simulink model "QUAD_EULER_MPC_SMC"  (R2024b)
settings: Solver=VariableStepAuto  StartTime=0.0  StopTime=10.0  RelTol=1e-3
values from neighbouring files (symbols this model uses):
  F1 = F1 + 2*(PSI_I'*C'*Q_z*C*PHI_I)    [Setup_MPC_SMC_Drone.m]
  F1_xy = F1_xy + 2*(PSI_xy_I'*C_xy'*Q_xy*C_xy*PHI_xy_I)    [Setup_MPC_SMC_Drone.m]
  F2 = F2 - 2*(PSI_I'*C'*Q_z*pi_n)    [Setup_MPC_SMC_Drone.m]
  F2_xy = F2_xy - 2*(PSI_xy_I'*C_xy'*Q_xy*pi_n)    [Setup_MPC_SMC_Drone.m]
  F3 = F3 - 2*(pi_nu'*Qt_z)    [Setup_MPC_SMC_Drone.m]
  F3_xy = F3_xy - 2*(pi_nu'*R_xy)    [Setup_MPC_SMC_Drone.m]
  F4 = F4 + 2*(PSI_I'*C'*Qt_z*C*SumG)    [Setup_MPC_SMC_Drone.m]
  g = 9.81    [Setup_MPC_SMC_Drone.m]
  G = [0;-g]    [Setup_MPC_SMC_Drone.m]
  H = H + 2*(PSI_I'*C'*Q_z*C*PSI_I + pi_nu'*Qt_z*pi_nu)    [Setup_MPC_SMC_Drone.m]
  H_xy = H_xy + 2*(PSI_xy_I'*C_xy'*Q_xy*C_xy*PSI_xy_I + pi_nu'*R_xy*pi_nu)    [Setup_MPC_SMC_Drone.m]
  J = diag([Jxx Jyy Jzz])    [Setup_MPC_SMC_Drone.m]
  m = 1.121    [Setup_MPC_SMC_Drone.m]
  N = 10    [Setup_MPC_SMC_Drone.m]
  N_xy = 10    [Setup_MPC_SMC_Drone.m]
  ny = size(C,1)    [Setup_MPC_SMC_Drone.m]
  ny_xy = size(C_xy,1)    [Setup_MPC_SMC_Drone.m]
  u_des = 0    [Setup_MPC_SMC_Drone.m]
  u_des_xy = [0;0]    [Setup_MPC_SMC_Drone.m]
undefined symbols (not defined in the file or in its folder): nu
libraries: matrix_library x1, aerolibutil x1
settings Model: Creator=Jorge  LastModifiedBy=Jorge

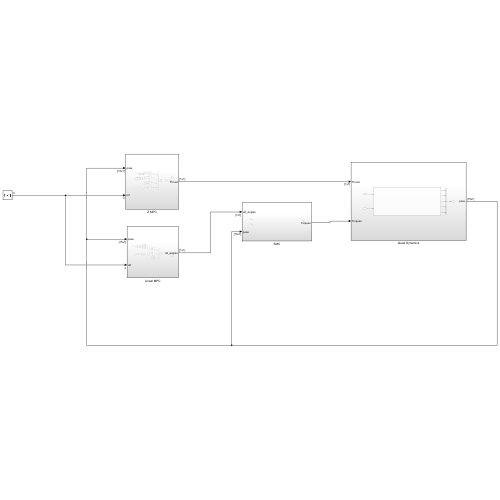
[thumbnail: Simulink's stored preview of the top-level diagram]
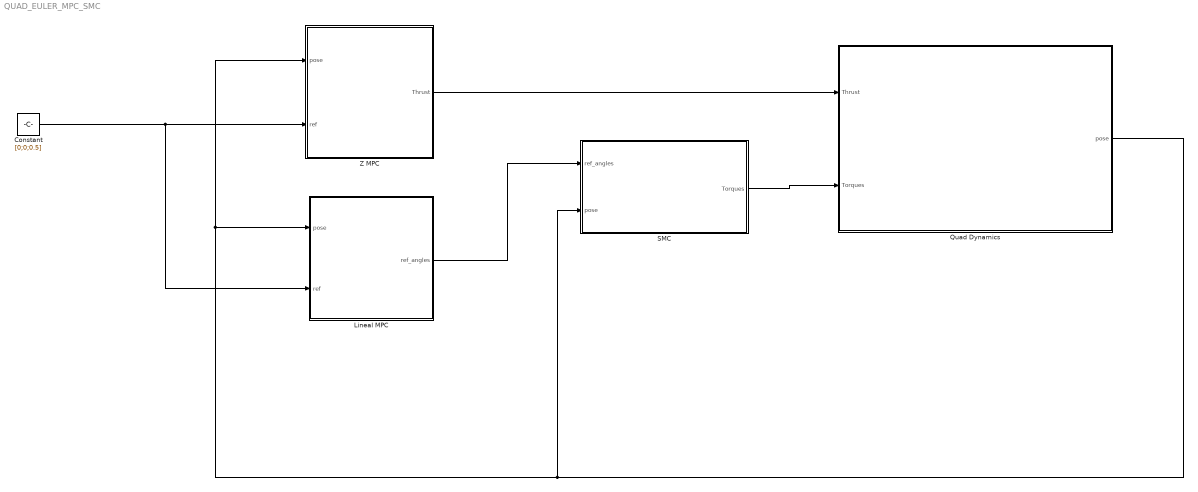
== system QUAD_EULER_MPC_SMC ==
  Constant : Constant  Value=[0;0;0.5]
  Lineal MPC : Subsystem
  Quad Dynamics : Subsystem
  SMC : Subsystem
  Z MPC : Subsystem
  wires:
  Quad Dynamics/1(pose) -> SMC/2(pose), Lineal MPC/1(pose), Z MPC/1(pose)
  Z MPC/1(Thrust) -> Quad Dynamics/1(Thrust)
  Constant/1 -> Lineal MPC/2(ref), Z MPC/2(ref)
  Lineal MPC/1(ref_angles) -> SMC/1(ref_angles)
  SMC/1(Torques) -> Quad Dynamics/2(Torques)

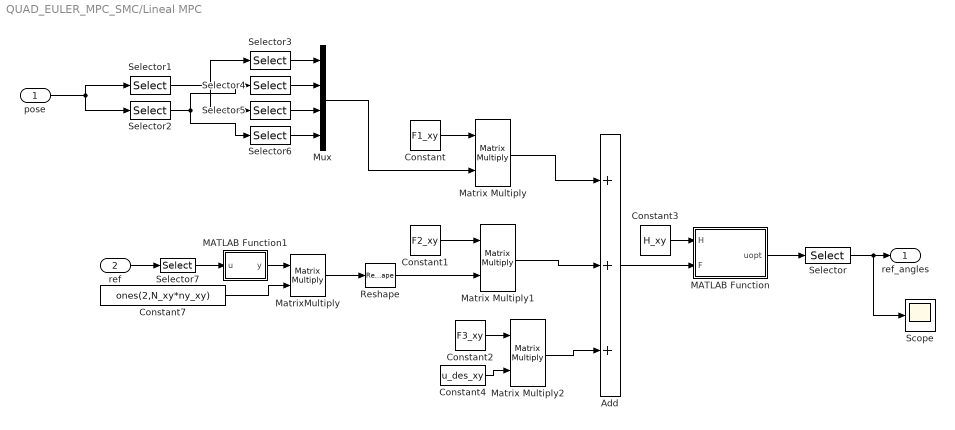
== system QUAD_EULER_MPC_SMC/Lineal MPC ==
  pose : Inport
  ref : Inport  Port=2
  Add : Sum  Inputs=+++
  Constant : Constant  Value=F1_xy
  Constant1 : Constant  Value=F2_xy
  Constant2 : Constant  Value=F3_xy
  Constant3 : Constant  Value=H_xy
  Constant4 : Constant  Value=u_des_xy
  Constant7 : Constant  Value=ones(2,N_xy*ny_xy)
  MATLAB Function : MATLAB Function  TreatAsAtomicUnit=on
  MATLAB Function1 : MATLAB Function  TreatAsAtomicUnit=on
  Matrix Multiply : Product  Multiplication=Matrix(*)
  Matrix Multiply1 : Product  Multiplication=Matrix(*)
  Matrix Multiply2 : Product  Multiplication=Matrix(*)
  MatrixMultiply : Product  Multiplication=Matrix(*)
  Mux : Mux
  Reshape : Reshape  OutputDimensionality=Customize  OutputDimensions=[N_xy*ny_xy,1]
  Scope : Scope
  Selector : Selector  InputPortWidth=20  IndexOptions=Index vector (dialog)  Indices=1  OutputSizes=1
  Selector1 : Selector  InputPortWidth=15  IndexOptions=Index vector (dialog)  Indices=[1 2]  OutputSizes=1
  Selector2 : Selector  InputPortWidth=15  IndexOptions=Index vector (dialog)  Indices=[4 5]  OutputSizes=1
  Selector3 : Selector  InputPortWidth=2  IndexOptions=Index vector (dialog)  Indices=1  OutputSizes=1
  Selector4 : Selector  InputPortWidth=2  IndexOptions=Index vector (dialog)  Indices=1  OutputSizes=1
  Selector5 : Selector  InputPortWidth=2  IndexOptions=Index vector (dialog)  Indices=2  OutputSizes=1
  Selector6 : Selector  InputPortWidth=2  IndexOptions=Index vector (dialog)  Indices=1  OutputSizes=1
  Selector7 : Selector  InputPortWidth=3  IndexOptions=Index vector (dialog)  Indices=[1:2]  OutputSizes=1
  ref_angles : Outport
  wires:
  Constant3/1 -> MATLAB Function/1(H)
  Add/1 -> MATLAB Function/2(F)
  MATLAB Function/1(uopt) -> Selector/1
  Selector/1 -> Scope/1, ref_angles/1
  pose/1 -> Selector2/1, Selector1/1
  Selector1/1 -> Selector3/1, Selector5/1
  Selector2/1 -> Selector4/1, Selector6/1
  Selector3/1 -> Mux/1
  Selector4/1 -> Mux/2
  Selector5/1 -> Mux/3
  Selector6/1 -> Mux/4
  Constant/1 -> Matrix Multiply/1
  Mux/1 -> Matrix Multiply/2
  Matrix Multiply/1 -> Add/1
  Matrix Multiply1/1 -> Add/2
  Constant1/1 -> Matrix Multiply1/1
  Constant7/1 -> MatrixMultiply/2
  ref/1 -> Selector7/1
  MatrixMultiply/1 -> Reshape/1
  Reshape/1 -> Matrix Multiply1/2
  Matrix Multiply2/1 -> Add/3
  Constant2/1 -> Matrix Multiply2/1
  Constant4/1 -> Matrix Multiply2/2
  Selector7/1 -> MATLAB Function1/1(u)
  MATLAB Function1/1(y) -> MatrixMultiply/1

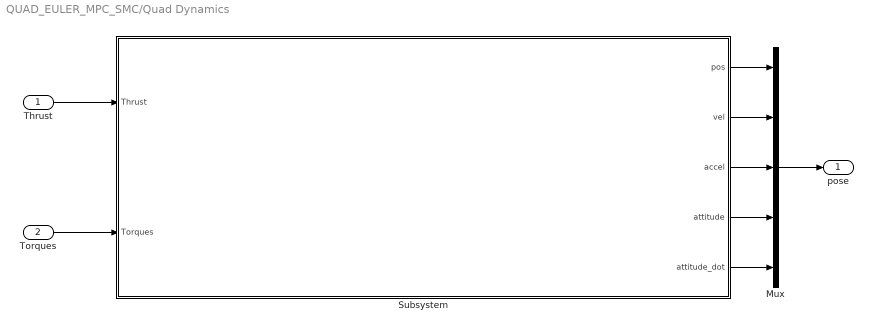
== system QUAD_EULER_MPC_SMC/Quad Dynamics ==
  Thrust : Inport
  Torques : Inport  Port=2
  Mux : Mux  Inputs=5
  Subsystem : Subsystem
  pose : Outport
  wires:
  Subsystem/1(pos) -> Mux/1
  Subsystem/2(vel) -> Mux/2
  Subsystem/3(accel) -> Mux/3
  Subsystem/4(attitude) -> Mux/4
  Subsystem/5(attitude_dot) -> Mux/5
  Thrust/1 -> Subsystem/1(Thrust)
  Torques/1 -> Subsystem/2(Torques)
  Mux/1 -> pose/1

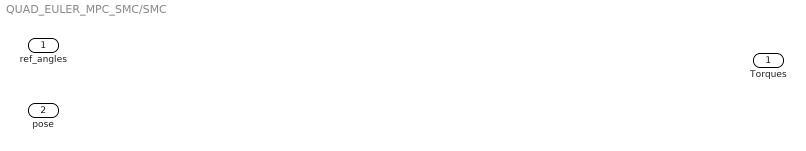
== system QUAD_EULER_MPC_SMC/SMC ==
  ref_angles : Inport
  pose : Inport  Port=2
  Torques : Outport

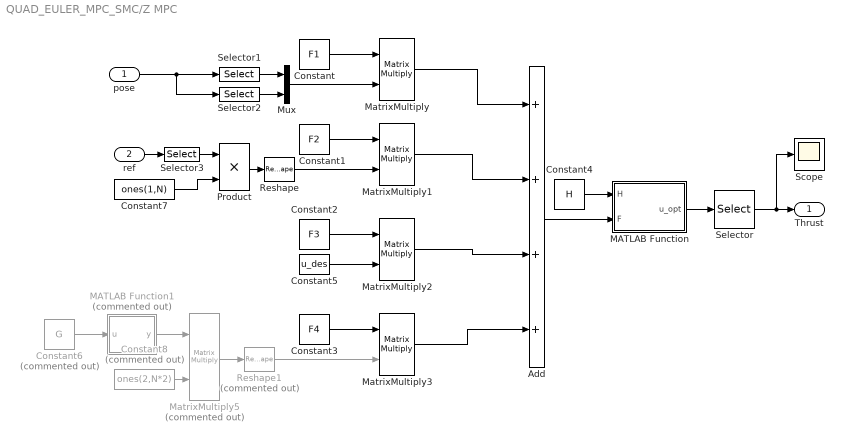
== system QUAD_EULER_MPC_SMC/Z MPC ==
  pose : Inport
  ref : Inport  Port=2
  Add : Sum  Inputs=++++
  Constant : Constant  Value=F1
  Constant1 : Constant  Value=F2
  Constant2 : Constant  Value=F3
  Constant3 : Constant  Value=F4
  Constant4 : Constant  Value=H
  Constant5 : Constant  Value=u_des
  Constant6 : Constant  Commented=on  Value=G
  Constant7 : Constant  Value=ones(1,N)
  Constant8 : Constant  Commented=on  Value=ones(2,N*2)
  MATLAB Function : MATLAB Function  TreatAsAtomicUnit=on
  MATLAB Function1 : MATLAB Function  Commented=on  TreatAsAtomicUnit=on
  MatrixMultiply{,1..3} (4 alike) : Product  Multiplication=Matrix(*)
  MatrixMultiply5 : Product  Commented=on  Multiplication=Matrix(*)
  Mux : Mux  Inputs=2
  Product : Product
  Reshape : Reshape  OutputDimensionality=Customize  OutputDimensions=[N*ny,1]
  Reshape1 : Reshape  Commented=on  OutputDimensionality=Customize  OutputDimensions=[2*N,1]
  Scope : Scope
  Selector : Selector  InputPortWidth=N*nu  IndexOptions=Index vector (dialog)  Indices=1  OutputSizes=1
  Selector1 : Selector  InputPortWidth=15  IndexOptions=Index vector (dialog)  Indices=3  OutputSizes=1
  Selector2 : Selector  InputPortWidth=15  IndexOptions=Index vector (dialog)  Indices=6  OutputSizes=1
  Selector3 : Selector  InputPortWidth=3  IndexOptions=Index vector (dialog)  Indices=3  OutputSizes=1
  Thrust : Outport
  wires:
  Add/1 -> MATLAB Function/2(F)
  Constant4/1 -> MATLAB Function/1(H)
  MATLAB Function/1(u_opt) -> Selector/1
  Selector/1 -> Scope/1, Thrust/1
  Constant/1 -> MatrixMultiply/1
  MatrixMultiply/1 -> Add/1
  MatrixMultiply1/1 -> Add/2
  MatrixMultiply2/1 -> Add/3
  MatrixMultiply3/1 -> Add/4
  Mux/1 -> MatrixMultiply/2
  Selector2/1 -> Mux/2
  Selector1/1 -> Mux/1
  pose/1 -> Selector2/1, Selector1/1
  Constant1/1 -> MatrixMultiply1/1
  Constant5/1 -> MatrixMultiply2/2
  Constant2/1 -> MatrixMultiply2/1
  ref/1 -> Selector3/1
  Constant7/1 -> Product/2
  Selector3/1 -> Product/1
  Product/1 -> Reshape/1
  Reshape/1 -> MatrixMultiply1/2
  Constant8/1 -> MatrixMultiply5/2
  Constant6/1 -> MATLAB Function1/1(u)
  MatrixMultiply5/1 -> Reshape1/1
  Reshape1/1 -> MatrixMultiply3/2
  Constant3/1 -> MatrixMultiply3/1
  MATLAB Function1/1(y) -> MatrixMultiply5/1

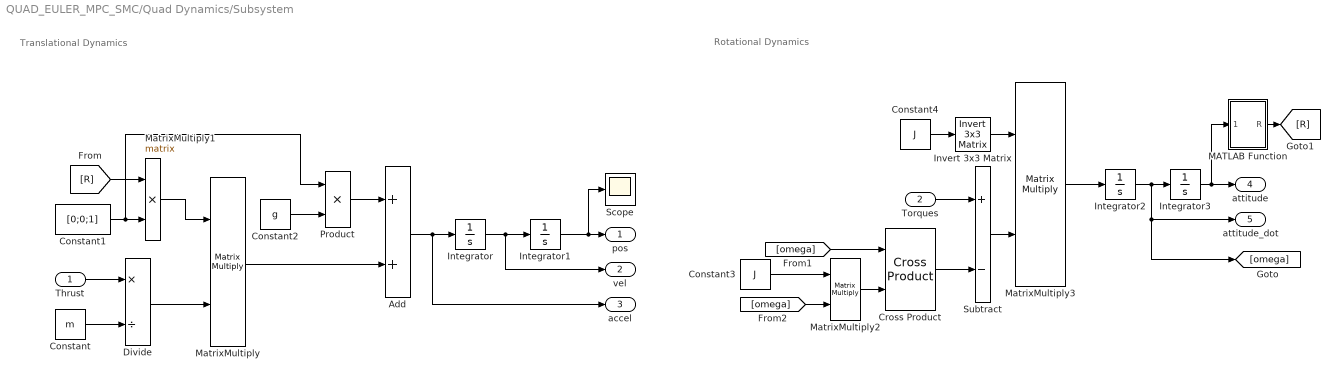
== system QUAD_EULER_MPC_SMC/Quad Dynamics/Subsystem ==
  note: Rotational Dynamics
  note: Translational Dynamics
  Thrust : Inport
  Torques : Inport  Port=2
  Add : Sum
  Constant : Constant  Value=m
  Constant1 : Constant  Value=[0;0;1]
  Constant2 : Constant  Value=g
  Constant3 : Constant  Value=J
  Constant4 : Constant  Value=J
  Cross Product : matrix_library/Cross Product
  Divide : Product  Inputs=*/
  Integrator{,1..3} (4 alike) : Integrator
  Invert 3x3 Matrix : aerolibutil/Invert  3x3 Matrix
  MATLAB Function : MATLAB Function  TreatAsAtomicUnit=on
  MatrixMultiply{,1..3} (4 alike) : Product  Multiplication=Matrix(*)
  Product : Product
  Scope : Scope
  Subtract : Sum  Inputs=+-
  pos : Outport
  vel : Outport  Port=2
  accel : Outport  Port=3
  attitude : Outport  Port=4
  attitude_dot : Outport  Port=5
  wires:
  Constant/1 -> Divide/2
  MatrixMultiply1/1 -> MatrixMultiply/1
  Integrator2/1 -> [omega], attitude_dot/1, Integrator3/1
  Constant2/1 -> Product/2
  Integrator1/1 -> Scope/1, pos/1
  Integrator/1 -> vel/1, Integrator1/1
  Constant4/1 -> Invert 3x3 Matrix/1
  [omega] -> Cross Product/1
  Constant3/1 -> MatrixMultiply2/1
  [omega] -> MatrixMultiply2/2
  Cross Product/1 -> Subtract/2
  Divide/1 -> MatrixMultiply/2
  Torques/1 -> Subtract/1
  [R] -> MatrixMultiply1/1
  MatrixMultiply/1 -> Add/2
  Integrator3/1 -> MATLAB Function/1(att), attitude/1
  MATLAB Function/1(R) -> [R]
  Constant1/1 -> Product/1, MatrixMultiply1/2
  MatrixMultiply3/1 -> Integrator2/1
  Add/1 -> accel/1, Integrator/1
  MatrixMultiply2/1 -> Cross Product/2
  Subtract/1 -> MatrixMultiply3/2
  Thrust/1 -> Divide/1
  Product/1 -> Add/1
  Invert 3x3 Matrix/1 -> MatrixMultiply3/1

== matlab function QUAD_EULER_MPC_SMC/Lineal MPC/MATLAB Function ==
  data: H input; uopt output; F input
function uopt = fcn(H,F)

uopt = -H\F;

== matlab function QUAD_EULER_MPC_SMC/Z MPC/MATLAB Function1 ==
  data: u input; y output
function y = fcn(u)

y = [u(1) u(2)];

== matlab function QUAD_EULER_MPC_SMC/Quad Dynamics/Subsystem/MATLAB Function ==
  data: att input; R output
function R = fcn(att)
phi = att(1);
theta = att(2);
psi = att(3);

R = [
cos(psi)*cos(theta), cos(psi)*sin(theta)*sin(phi) - cos(phi)*sin(psi), cos(psi)*cos(phi)*sin(theta)+sin(phi)*sin(psi);
cos(theta)*sin(psi), sin(psi)*sin(phi)*sin(theta) + cos(phi)*cos(psi), sin(psi)*cos(phi)*sin(theta)-cos(psi)*sin(phi);
-sin(theta),cos(theta)*sin(phi), cos(phi)*cos(theta);
];

== matlab function QUAD_EULER_MPC_SMC/Lineal MPC/MATLAB Function1 ==
  data: u input; y output
function y = fcn(u)

y = [u(1),u(2)];

== matlab function QUAD_EULER_MPC_SMC/Z MPC/MATLAB Function ==
  data: H input; u_opt output; F input
function u_opt = fcn(H,F)

u_opt = -H\F;
